simulink model "sim_linear_control_y"  (R2018a)
settings: Solver=ode3  StartTime=0.0  StopTime=10  FixedStep=0.001  RelTol=1e-3
values from neighbouring files (symbols this model uses):
  CA = C*A    [lin_control_error.m]    (also in lin_control_psi.m; lin_control_y.m)
  fc = 0.5    [lin_control_error.m]    (also in lin_control_y.m)
  invCB = pinv(C*B)    [lin_control_error.m]    (also in lin_control_psi.m; lin_control_y.m)
  Kb_Vy = 8    [lin_control_y.m]
  Kb_y = 2    [lin_control_y.m]
  Vx = 30    [lin_control_error.m]    (also in lin_control_psi.m = 8.33333333333; lin_control_y.m = 8.33333333333)
settings Model: Creator=E183308  LastModifiedBy=E183308

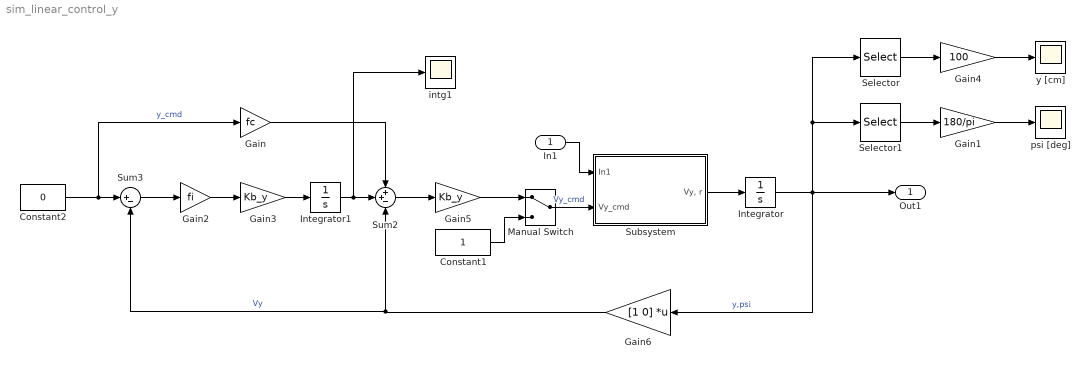
== system sim_linear_control_y ==
  In1 : Inport
  Constant1 : Constant
  Constant2 : Constant  Value=0
  Gain : Gain  Gain=fc
  Gain1 : Gain  Gain=180/pi
  Gain2 : Gain  Gain=fi
  Gain3 : Gain  Gain=Kb_y
  Gain4 : Gain  Gain=100
  Gain5 : Gain  Gain=Kb_y
  Gain6 : Gain  Gain=[1 0]  Multiplication=Matrix(K*u)
  Integrator : Integrator
  Integrator1 : Integrator
  Manual Switch : ManualSwitch
  Selector : Selector  InputPortWidth=2  IndexOptions=Index vector (dialog)  Indices=1  OutputSizes=1
  Selector1 : Selector  InputPortWidth=2  IndexOptions=Index vector (dialog)  Indices=1  OutputSizes=1
  Subsystem : Subsystem
  Sum2 : Sum  Inputs=++-
  Sum3 : Sum  Inputs=|+-
  intg1 : Scope
  psi [deg] : Scope
  y [cm] : Scope
  Out1 : Outport
  wires:
  Constant1/1 -> Manual Switch/2
  Gain5/1 -> Manual Switch/1
  Subsystem/1("Vy, r") -> Integrator/1
  In1/1 -> Subsystem/1(In1)
  Manual Switch/1 -> Subsystem/2(Vy_cmd)  "Vy_cmd"
  Integrator/1 -> Selector1/1, Selector/1, Out1/1, Gain6/1  "y,psi"
  Selector/1 -> Gain4/1
  Selector1/1 -> Gain1/1
  Gain1/1 -> psi [deg]/1
  Constant2/1 -> Gain/1, Sum3/1  "y_cmd"
  Sum3/1 -> Gain2/1
  Gain2/1 -> Gain3/1
  Gain3/1 -> Integrator1/1
  Integrator1/1 -> intg1/1, Sum2/2
  Gain/1 -> Sum2/1
  Sum2/1 -> Gain5/1
  Gain6/1 -> Sum3/2, Sum2/3  "Vy"
  Gain4/1 -> y [cm]/1

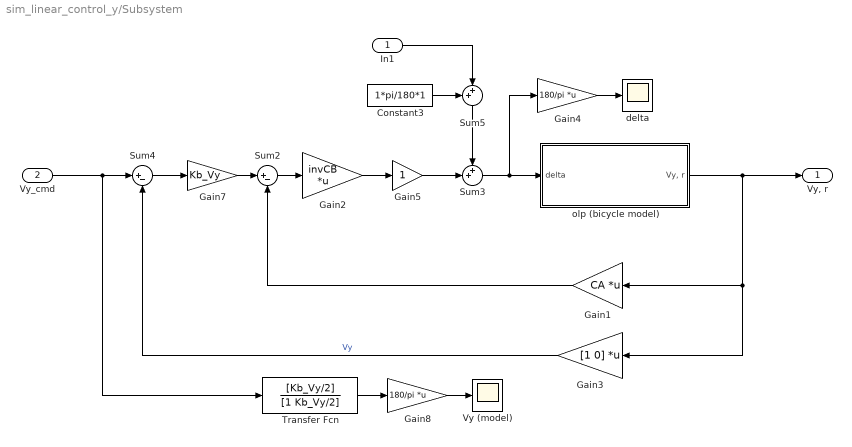
== system sim_linear_control_y/Subsystem ==
  In1 : Inport
  Vy_cmd : Inport  Port=2
  Constant3 : Constant  Value=1*pi/180*1
  Gain1 : Gain  Gain=CA  Multiplication=Matrix(K*u)
  Gain2 : Gain  Gain=invCB  Multiplication=Matrix(K*u)
  Gain3 : Gain  Gain=[1 0]  Multiplication=Matrix(K*u)
  Gain4 : Gain  Gain=180/pi  Multiplication=Matrix(K*u)
  Gain5 : Gain
  Gain7 : Gain  Gain=Kb_Vy
  Gain8 : Gain  Gain=180/pi  Multiplication=Matrix(K*u)
  Sum2 : Sum  Inputs=|+-
  Sum3 : Sum  Inputs=++|
  Sum4 : Sum  Inputs=|+-
  Sum5 : Sum  Inputs=++|
  Transfer Fcn : TransferFcn  Numerator=[Kb_Vy/2]  Denominator=[1 Kb_Vy/2]
  Vy (model) : Scope
  delta : Scope
  olp (bicycle model) : Subsystem
  "Vy, r" : Outport
  wires:
  Gain4/1 -> delta/1
  Vy_cmd/1 -> Transfer Fcn/1, Sum4/1
  Gain3/1 -> Sum4/2  "Vy"
  Transfer Fcn/1 -> Gain8/1
  Gain8/1 -> Vy (model)/1
  Gain2/1 -> Gain5/1
  Sum2/1 -> Gain2/1
  Sum3/1 -> Gain4/1, olp (bicycle model)/1(delta)
  Sum4/1 -> Gain7/1
  Constant3/1 -> Sum5/1
  Sum5/1 -> Sum3/1
  Gain1/1 -> Sum2/2
  Gain7/1 -> Sum2/1
  In1/1 -> Sum5/2
  olp (bicycle model)/1("Vy, r") -> Gain3/1, Gain1/1, "Vy, r"/1
  Gain5/1 -> Sum3/2

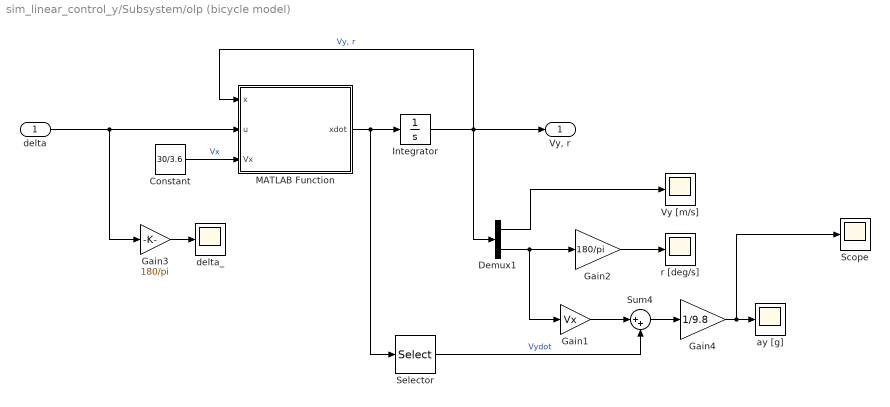
== system sim_linear_control_y/Subsystem/olp (bicycle model) ==
  delta : Inport
  Constant : Constant  Value=30/3.6
  Demux1 : Demux  Outputs=2
  Gain1 : Gain  Gain=Vx
  Gain2 : Gain  Gain=180/pi
  Gain3 : Gain  Gain=180/pi
  Gain4 : Gain  Gain=1/9.8
  Integrator : Integrator  InitialCondition=[0;0]
  MATLAB Function : MATLAB Function  TreatAsAtomicUnit=on
  Scope : Scope
  Selector : Selector  InputPortWidth=2  IndexOptions=Index vector (dialog)  Indices=1  OutputSizes=1
  Sum4 : Sum  Inputs=|++
  Vy [m/s] : Scope
  ay [g] : Scope
  delta_ : Scope
  r [deg/s] : Scope
  "Vy, r" : Outport
  wires:
  Gain2/1 -> r [deg/s]/1
  Demux1/2 -> Gain1/1, Gain2/1
  Integrator/1 -> MATLAB Function/1(x), "Vy, r"/1, Demux1/1  "Vy, r"
  Gain3/1 -> delta_/1
  delta/1 -> Gain3/1, MATLAB Function/2(u)
  Constant/1 -> MATLAB Function/3(Vx)  "Vx"
  MATLAB Function/1(xdot) -> Selector/1, Integrator/1
  Demux1/1 -> Vy [m/s]/1
  Gain1/1 -> Sum4/1
  Selector/1 -> Sum4/2  "Vydot"
  Sum4/1 -> Gain4/1
  Gain4/1 -> Scope/1, ay [g]/1

== matlab function sim_linear_control_y/Subsystem/olp (bicycle model)/MATLAB Function ==
  data: x input; u input; xdot output; Vx input
function xdot = dynamic_lin(x,u,Vx)

% sports sedan

m = 1724; % kg
Iz = 3400; % kg/m^2
a = 1.35; % m
b = 1.15; % m
Cf = 12*1e4; % N/rad
Cr = 175*1e3; % N/rad
mu = 0.5225;

% x = [vy r]
% u = delta

A = [-(Cf+Cr)/(m*Vx)  -(a*Cf-b*Cr)/(m*Vx)-Vx; 
    -(a*Cf-b*Cr)/(Iz*Vx) -(a^2*Cf+b^2*Cr)/(Iz*Vx)];

B = [Cf/m; a*Cf/Iz];

xdot = A*x + B*u;
